simulink model "HybridSimulinkModel"  (R2020a)
settings: Solver=VariableStepAuto  StartTime=0.0  StopTime=Days  RelTol=1e-3
values from neighbouring files (symbols this model uses):
  A_know = x(5)    [ObjPred.m]
  A_social = x(3)    [ObjPred.m]
  B_know = x(6)    [ObjPred.m]
  B_social = x(4)    [ObjPred.m]
  K = abs(x(19))    [ObjPred.m]
  k_equalizer = x(10)    [ObjPred.m]
  k_inp = x(24)    [ObjPred.m]
  k_p_hs = x(14)    [ObjPred.m]
  P_cog = x(17)    [ObjPred.m]
  T_cog = abs(x(18))    [ObjPred.m]
  T_emg = abs(x(23))    [ObjPred.m]
  T_I_Amb = x(26)    [ObjPred.m]
  T_I_Emg = x(28)    [ObjPred.m]
  T_I_hs = x(16)    [ObjPred.m]
  T_I_Med = x(30)    [ObjPred.m]
  T_in = abs(x(22))    [ObjPred.m]
  T_L_Amb = x(25)    [ObjPred.m]
  T_L_Emg = x(27)    [ObjPred.m]
  T_L_hs = x(15)    [ObjPred.m]
  T_L_Med = x(29)    [ObjPred.m]
  TI = x(9)    [ObjPred.m]
  time_delay = abs(x(7))    [ObjPred.m]
  TL = x(8)    [ObjPred.m]
  TN_p = x(11)    [ObjPred.m]
  wn_de = x(32)    [ObjPred.m]
  wn_h = x(21)    [ObjPred.m]
  wn_s = x(13)    [ObjPred.m]
  zn_de = x(31)    [ObjPred.m]
  zn_h = x(20)    [ObjPred.m]
  zn_s = x(12)    [ObjPred.m]
undefined symbols (not defined in the file or in its folder): fin_maxrate
libraries: simulink x5
settings Model: SimulationMode=accelerator  Creator=miad  LastModifiedBy=miad

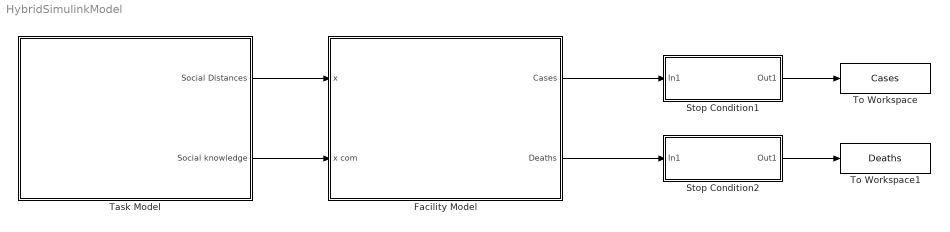
== system HybridSimulinkModel ==
  Facility Model : Subsystem
  Stop Condition1 : Subsystem
  Stop Condition2 : Subsystem
  Task Model : Subsystem
  To Workspace : ToWorkspace  VariableName=Cases  SampleTime=-1
      settings: Save2DSignal=2-D array (concatenate along first dimension)
  To Workspace1 : ToWorkspace  VariableName=Deaths  SampleTime=-1
      settings: Save2DSignal=2-D array (concatenate along first dimension)
  wires:
  Facility Model/1(Cases) -> Stop Condition1/1(In1)
  Stop Condition1/1(Out1) -> To Workspace/1
  Facility Model/2(Deaths) -> Stop Condition2/1(In1)
  Task Model/1(Social Distances) -> Facility Model/1(x)
  Task Model/2(Social knowledge) -> Facility Model/2(x com)
  Stop Condition2/1(Out1) -> To Workspace1/1

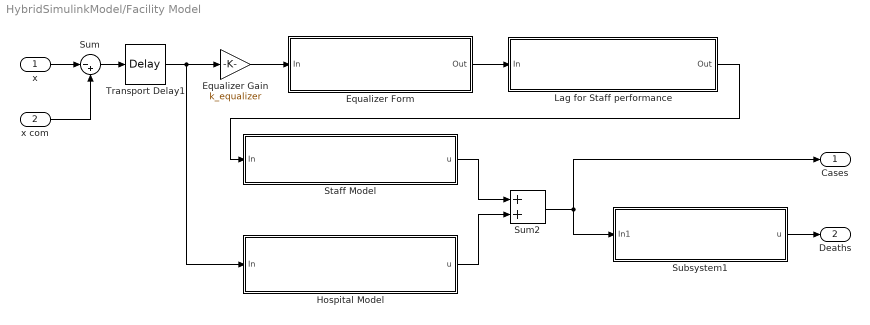
== system HybridSimulinkModel/Facility Model ==
  x : Inport
  x com : Inport  Port=2
  Equalizer Gain : Gain  Gain=k_equalizer
  Equalizer Form : Subsystem
  Hospital Model : Subsystem
  Lag for Staff performance : Subsystem
  Staff Model : Subsystem
  Subsystem1 : Subsystem
  Sum : Sum  Inputs=|-+
  Sum2 : Sum
  Transport Delay1 : TransportDelay  DelayTime=time_delay
  Cases : Outport  VectorParamsAs1DForOutWhenUnconnected=off
  Deaths : Outport  Port=2  VectorParamsAs1DForOutWhenUnconnected=off
  wires:
  Equalizer Gain/1 -> Equalizer Form/1(In)
  x com/1 -> Sum/2
  x/1 -> Sum/1
  Sum/1 -> Transport Delay1/1
  Transport Delay1/1 -> Hospital Model/1(In), Equalizer Gain/1
  Equalizer Form/1(Out) -> Lag for Staff performance/1(In)
  Subsystem1/1(u) -> Deaths/1
  Lag for Staff performance/1(Out) -> Staff Model/1(In)
  Staff Model/1(u) -> Sum2/1
  Hospital Model/1(u) -> Sum2/2
  Sum2/1 -> Cases/1, Subsystem1/1(In1)

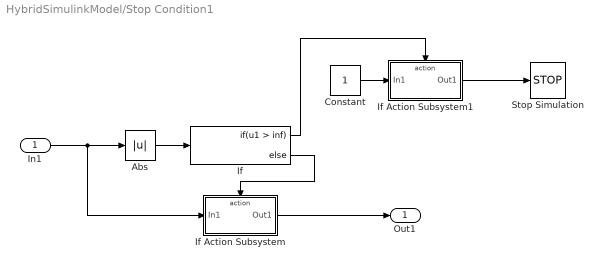
== system HybridSimulinkModel/Stop Condition1 ==
  In1 : Inport
  Abs : Abs
  Constant : Constant
  If : If  IfExpression=u1 > inf
  If Action Subsystem : Subsystem  TreatAsAtomicUnit=on
  If Action Subsystem1 : Subsystem  TreatAsAtomicUnit=on
  Stop Simulation : Stop
  Out1 : Outport
  wires:
  If Action Subsystem/1(Out1) -> Out1/1
  In1/1 -> If Action Subsystem/1(In1), Abs/1
  If/2 -> If Action Subsystem/Action
  Abs/1 -> If/1
  If/1 -> If Action Subsystem1/Action
  If Action Subsystem1/1(Out1) -> Stop Simulation/1
  Constant/1 -> If Action Subsystem1/1(In1)

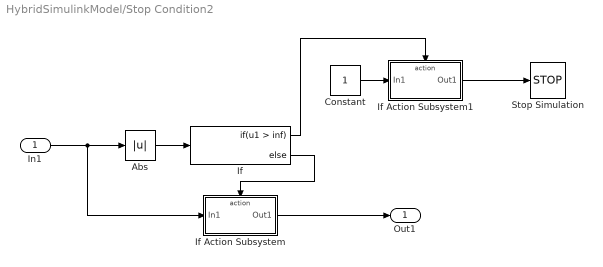
== system HybridSimulinkModel/Stop Condition2 ==
  In1 : Inport
  Abs : Abs
  Constant : Constant
  If : If  IfExpression=u1 > inf
  If Action Subsystem : Subsystem  TreatAsAtomicUnit=on
  If Action Subsystem1 : Subsystem  TreatAsAtomicUnit=on
  Stop Simulation : Stop
  Out1 : Outport
  wires:
  Constant/1 -> If Action Subsystem1/1(In1)
  If Action Subsystem1/1(Out1) -> Stop Simulation/1
  If/1 -> If Action Subsystem1/Action
  Abs/1 -> If/1
  If/2 -> If Action Subsystem/Action
  In1/1 -> Abs/1, If Action Subsystem/1(In1)
  If Action Subsystem/1(Out1) -> Out1/1

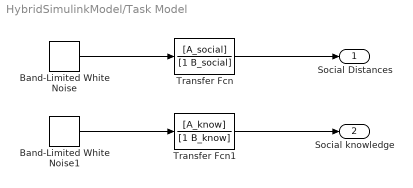
== system HybridSimulinkModel/Task Model ==
  Band-Limited White Noise : simulink/Sources/Band-Limited White Noise  Cov=Power_social  Ts=0.1  seed=[23341]
  Band-Limited White Noise1 : simulink/Sources/Band-Limited White Noise  Cov=Power_know  Ts=0.1  seed=[23341]
  Transfer Fcn : TransferFcn  Numerator=[A_social]  Denominator=[1 B_social]
  Transfer Fcn1 : TransferFcn  Numerator=[A_know]  Denominator=[1 B_know]
  Social Distances : Outport
  Social knowledge : Outport  Port=2
  wires:
  Band-Limited White Noise/1 -> Transfer Fcn/1
  Band-Limited White Noise1/1 -> Transfer Fcn1/1
  Transfer Fcn/1 -> Social Distances/1
  Transfer Fcn1/1 -> Social knowledge/1

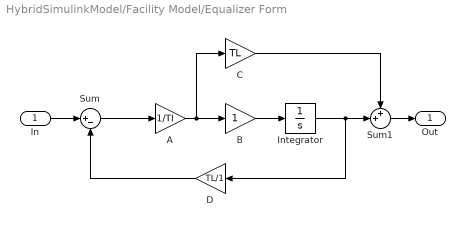
== system HybridSimulinkModel/Facility Model/Equalizer Form ==
  In : Inport
  A : Gain  Gain=1/TI
  B : Gain
  C : Gain  Gain=TL
  D : Gain  Gain=TL/1
  Integrator : Integrator
  Sum : Sum  Inputs=|+-
  Sum1 : Sum  Inputs=++|
  Out : Outport  VectorParamsAs1DForOutWhenUnconnected=off
  wires:
  Sum1/1 -> Out/1
  Sum/1 -> A/1
  In/1 -> Sum/1
  C/1 -> Sum1/1
  D/1 -> Sum/2
  Integrator/1 -> Sum1/2, D/1
  B/1 -> Integrator/1
  A/1 -> C/1, B/1

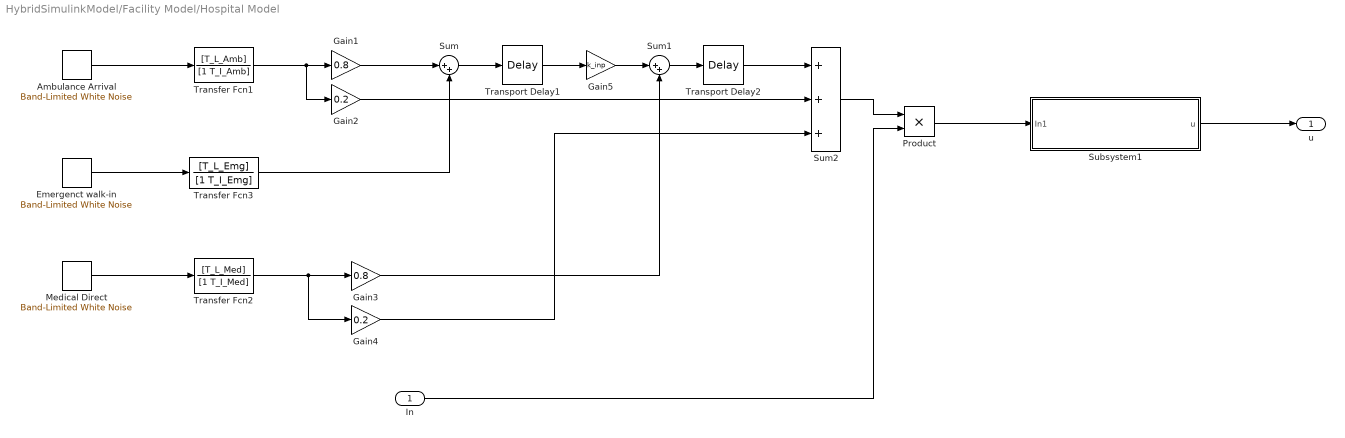
== system HybridSimulinkModel/Facility Model/Hospital Model ==
  In : Inport
  Ambulance Arrival : simulink/Sources/Band-Limited White Noise  Cov=Power_Amb  Ts=0.1  seed=[23341]
  Emergenct walk-in : simulink/Sources/Band-Limited White Noise  Cov=Power_Emg  Ts=0.1  seed=[23341]
  Gain1 : Gain  Gain=0.8
  Gain2 : Gain  Gain=0.2
  Gain3 : Gain  Gain=0.8
  Gain4 : Gain  Gain=0.2
  Gain5 : Gain  Gain=k_inp
  Medical Direct : simulink/Sources/Band-Limited White Noise  Cov=Power_Med  Ts=0.1  seed=[23341]
  Product : Product
  Subsystem1 : Subsystem
  Sum : Sum  Inputs=|++
  Sum1 : Sum  Inputs=|++
  Sum2 : Sum  Inputs=+++
  Transfer Fcn1 : TransferFcn  Numerator=[T_L_Amb]  Denominator=[1 T_I_Amb]
  Transfer Fcn2 : TransferFcn  Numerator=[T_L_Med]  Denominator=[1 T_I_Med]
  Transfer Fcn3 : TransferFcn  Numerator=[T_L_Emg]  Denominator=[1 T_I_Emg]
  Transport Delay1 : TransportDelay  DelayTime=T_emg
  Transport Delay2 : TransportDelay  DelayTime=T_in
  u : Outport  VectorParamsAs1DForOutWhenUnconnected=off
  wires:
  Transfer Fcn1/1 -> Gain2/1, Gain1/1
  Transfer Fcn2/1 -> Gain4/1, Gain3/1
  Gain1/1 -> Sum/1
  Transfer Fcn3/1 -> Sum/2
  Sum/1 -> Transport Delay1/1
  Transport Delay1/1 -> Gain5/1
  Gain5/1 -> Sum1/1
  Gain3/1 -> Sum1/2
  Sum1/1 -> Transport Delay2/1
  Transport Delay2/1 -> Sum2/1
  Medical Direct/1 -> Transfer Fcn2/1
  Emergenct walk-in/1 -> Transfer Fcn3/1
  Ambulance Arrival/1 -> Transfer Fcn1/1
  Gain2/1 -> Sum2/2
  Product/1 -> Subsystem1/1(In1)
  Sum2/1 -> Product/1
  Gain4/1 -> Sum2/3
  In/1 -> Product/2
  Subsystem1/1(u) -> u/1

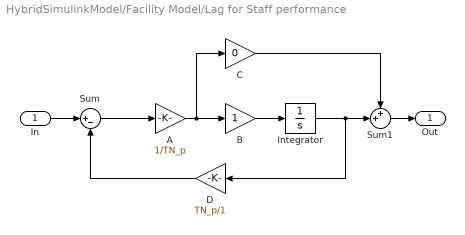
== system HybridSimulinkModel/Facility Model/Lag for Staff performance ==
  In : Inport
  A : Gain  Gain=1/TN_p
  B : Gain
  C : Gain  Gain=0
  D : Gain  Gain=TN_p/1
  Integrator : Integrator
  Sum : Sum  Inputs=|+-
  Sum1 : Sum  Inputs=++|
  Out : Outport  VectorParamsAs1DForOutWhenUnconnected=off
  wires:
  In/1 -> Sum/1
  Sum1/1 -> Out/1
  A/1 -> C/1, B/1
  B/1 -> Integrator/1
  Integrator/1 -> Sum1/2, D/1
  Sum/1 -> A/1
  C/1 -> Sum1/1
  D/1 -> Sum/2

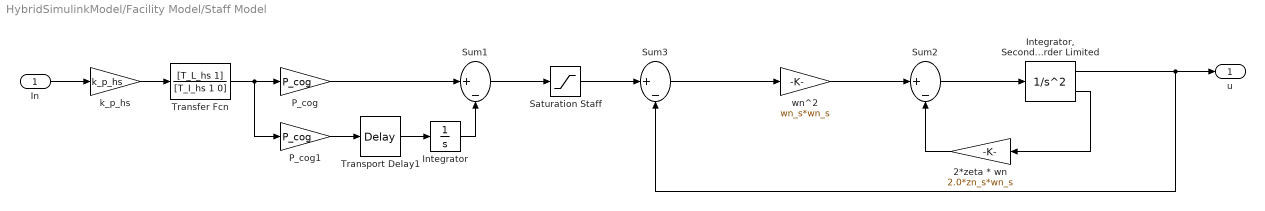
== system HybridSimulinkModel/Facility Model/Staff Model ==
  In : Inport
  2*zeta * wn : Gain  Gain=2.0*zn_s*wn_s  SaturateOnIntegerOverflow=on  OutDataTypeStr=Inherit: Same as input  ParamDataTypeStr=Inherit: Same as input
  Integrator : Integrator
  "Integrator, Second-Order Limited" : SecondOrderIntegrator  ICX=0  UpperLimitX=fin_max  LowerLimitX=fin_min  ICDXDT=0  UpperLimitDXDT=fin_maxrate  LowerLimitDXDT=-fin_maxrate
  P_cog : Gain  Gain=P_cog  SaturateOnIntegerOverflow=on  OutDataTypeStr=Inherit: Same as input  ParamDataTypeStr=Inherit: Same as input
  P_cog1 : Gain  Gain=P_cog  SaturateOnIntegerOverflow=on  OutDataTypeStr=Inherit: Same as input  ParamDataTypeStr=Inherit: Same as input
  Saturation Staff : Saturate  UpperLimit=K  LowerLimit=-K
  Sum1 : Sum  Inputs=|+-  InputSameDT=on  SaturateOnIntegerOverflow=on  OutDataTypeStr=Inherit: Same as first input
  Sum2 : Sum  Inputs=|+-  InputSameDT=on  SaturateOnIntegerOverflow=on  OutDataTypeStr=Inherit: Same as first input
  Sum3 : Sum  Inputs=|+-  InputSameDT=on  SaturateOnIntegerOverflow=on  OutDataTypeStr=Inherit: Same as first input
  Transfer Fcn : TransferFcn  Numerator=[T_L_hs 1]  Denominator=[T_I_hs 1 0]
  Transport Delay1 : TransportDelay  DelayTime=T_cog
  k_p_hs : Gain  Gain=k_p_hs  SaturateOnIntegerOverflow=on  OutDataTypeStr=Inherit: Same as input  ParamDataTypeStr=Inherit: Same as input
  wn^2 : Gain  Gain=wn_s*wn_s  SaturateOnIntegerOverflow=on  OutDataTypeStr=Inherit: Same as input  ParamDataTypeStr=Inherit: Same as input
  u : Outport  VectorParamsAs1DForOutWhenUnconnected=off
  wires:
  Sum2/1 -> "Integrator, Second-Order Limited"/1
  2*zeta * wn/1 -> Sum2/2
  Sum3/1 -> wn^2/1
  wn^2/1 -> Sum2/1
  "Integrator, Second-Order Limited"/1 -> Sum3/2, u/1
  "Integrator, Second-Order Limited"/2 -> 2*zeta * wn/1
  In/1 -> k_p_hs/1
  k_p_hs/1 -> Transfer Fcn/1
  Transfer Fcn/1 -> P_cog1/1, P_cog/1
  P_cog1/1 -> Transport Delay1/1
  Transport Delay1/1 -> Integrator/1
  Integrator/1 -> Sum1/2
  P_cog/1 -> Sum1/1
  Sum1/1 -> Saturation Staff/1
  Saturation Staff/1 -> Sum3/1

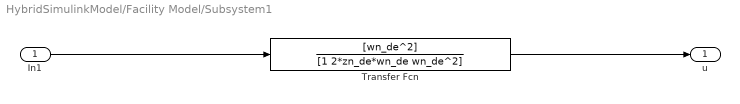
== system HybridSimulinkModel/Facility Model/Subsystem1 ==
  In1 : Inport
  Transfer Fcn : TransferFcn  Numerator=[wn_de^2]  Denominator=[1 2*zn_de*wn_de wn_de^2]
  u : Outport
  wires:
  In1/1 -> Transfer Fcn/1
  Transfer Fcn/1 -> u/1

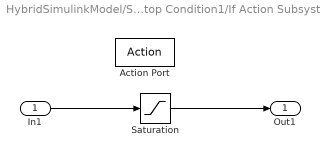
== system HybridSimulinkModel/Stop Condition1/If Action Subsystem ==
  In1 : Inport
  Action Port : ActionPort  ActionPortLabel=else
  Saturation : Saturate  UpperLimit=1e6  LowerLimit=0
  Out1 : Outport
  wires:
  In1/1 -> Saturation/1
  Saturation/1 -> Out1/1

== system HybridSimulinkModel/Stop Condition1/If Action Subsystem1 ==
  In1 : Inport
  Action Port : ActionPort  ActionPortLabel=if(u1 > inf)
  Out1 : Outport
  wires:
  In1/1 -> Out1/1

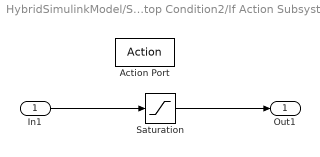
== system HybridSimulinkModel/Stop Condition2/If Action Subsystem ==
  In1 : Inport
  Action Port : ActionPort  ActionPortLabel=else
  Saturation : Saturate  UpperLimit=1e6  LowerLimit=0
  Out1 : Outport
  wires:
  In1/1 -> Saturation/1
  Saturation/1 -> Out1/1

== system HybridSimulinkModel/Stop Condition2/If Action Subsystem1 ==
  In1 : Inport
  Action Port : ActionPort  ActionPortLabel=if(u1 > inf)
  Out1 : Outport
  wires:
  In1/1 -> Out1/1

== system HybridSimulinkModel/Facility Model/Hospital Model/Subsystem1 ==
  In1 : Inport
  Transfer Fcn : TransferFcn  Numerator=[wn_h^2]  Denominator=[1 2*zn_h*wn_h wn_h^2]
  u : Outport
  wires:
  In1/1 -> Transfer Fcn/1
  Transfer Fcn/1 -> u/1
